simulink model "VBY_grid"  (R2024b)
settings: Solver=VariableStepAuto  StartTime=0.0  StopTime=24  MaxStep=0.33333333333333331  RelTol=1e-3  AbsTol=1e-3
values from neighbouring files (symbols this model uses):
  chargepower = 2E5    (= 200000)    [VBY_Script.m]
  terminalpower = 2E5    (= 200000)    [VBY_Script.m]
libraries: ee_lib x20, nesl_utility x16, fl_lib x10, simulink x8
settings Model: Creator=thoma  LastModifiedBy=thoma
settings SolverCC: AutoScaleAbsTol=off  DaesscMode=Robust
settings RTWCC: GenCodeOnly=on
settings SimscapeCC: SimscapeLogType=all

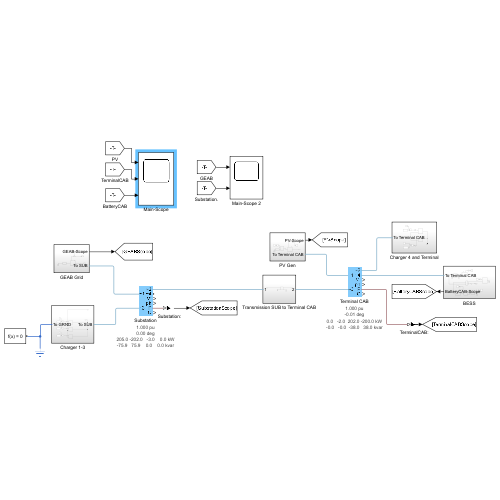
[thumbnail: Simulink's stored preview of the top-level diagram]
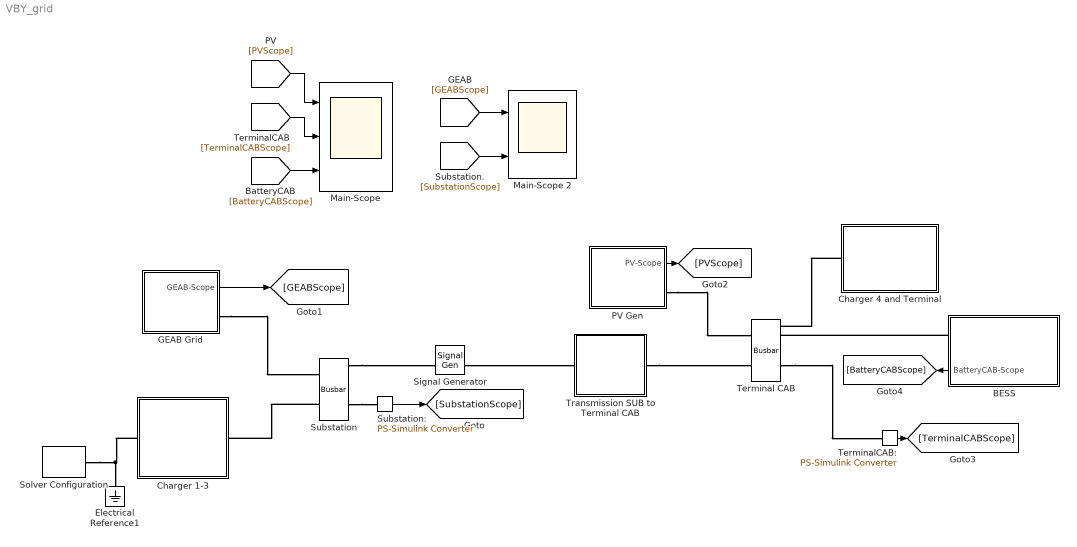
== system VBY_grid ==
  BESS : Subsystem
      settings: PortSchema="{\"entries\":[{\"content\":{\"sides\":[{\"content\":{\"connectorIds\":[\"LConn1\",\"Out1\"]},\"type\":\"ConnectorPlacement.EquallySpacedRectSide\",\"uuid\":\"78a52686-050b-473c-a829-dc142b2c03df\"},{\"content\":{\"side\":\"RIGHT\"},\"type\":\"ConnectorPlacement.EquallySpacedRectSide\",\"uuid\":\"16e0a1dc-1e2b-41fa-aa9e-07b8fe218401\"},{\"content\":{\"side\":\"TOP\"},\"type\":\"ConnectorPlacement.EquallySpacedRectSide\",\"uuid\":\"598e8960-ce00-4dd1-b062-18bc04a546a6\"}]},\"type\":\"ConnectorPlacement.EquallySpacedConnector\",\"uuid\":\"625199ba-0c11-4d67-98b2-801757f8b5e4\"}],\"packageUris\":[\"http://schema.mathworks.com/mf0/Connector/R2020b\"],\"version\":\"1.0\"}"
  Charger 1-3 : Subsystem
  Charger 4 and Terminal : Subsystem
  Electrical Reference1 : fl_lib/Electrical/Electrical Elements/Electrical Reference
  GEAB Grid : Subsystem
  Main-Scope : Scope  NumInputPorts=3
  Main-Scope 2 : Scope  NumInputPorts=2
  PV Gen : Subsystem
  Solver Configuration : nesl_utility/Solver Configuration  PhysicalDomain=network_engine_domain  SubClassName=solver  LeftPortType=input  RightPortType=generic  Tones=[]  Harmonics=[]  SimulateNoise=off  Profile=off  UseLocalSampling=off  EnableSwitchedLinearOptims=on  FrequencyDomain=off  UseCCode=off  RelTol=0.001  AbsTol=0.001  MinStep=1e-09  ToWorkspace=off  RevertToSquareIcSolve=off  NumHomotopyIterations=100  PhasorMode=off  PhasorModeNumHarmonics=1  ConsistencySolver=NEWTON_XTOL_AFTER_FTOL  IndexReductionMethod=DerivativeReplacement  DoDC=on  ResidualTolerance=1e-09  ConsistencyTolSource=GLOBAL  ConsistencyAbsTol=0.001  ConsistencyRelTol=0.001  ConsistencyTolFactor=0.0001  UseLocalSolver=off  LocalSolverChoice=NE_BACKWARD_EULER_ADVANCER  ResolveIndetEquations=on  FunctionEvalNumThread=1  LocalSolverSampleTime=0.001  DoFixedCost=off  MaxNonlinIter=3  MaxModeIter=2  ComputeImpulses=off  ImpulseIterations=2  LinearAlgebra=auto  LinearAlgebraNumThread=0  EquationFormulation=NE_FREQUENCY_TIME_EF  DelaysMemoryBudget=1024  AutomaticFiltering=on  FilteringTimeConstant=0.001  PartitionStorageMethod=AS_NEEDED  PartitionMemoryBudget=1024  PartitionMethod=ROBUST  MultibodyUseLocalSolver=off  MultibodyLocalSolverChoice=ODE1  MultibodyLocalSolverSampleTime=0.001
  Substation : ee_lib/Connectors & References/Busbar  Tag="1.000 pu\\n0.00 deg\\n205.0 -202.0   -3.0    0.0 kW\\n-75.9   75.9    0.0    0.0 kvar"  n_nodes=ee.enum.connectors.busbar_number_of_connections.four  VRated=11 kV  freq=50 Hz  show_ps=ee.enum.connectors.busbar_measurement.true
      settings: AttributesFormatString=%<Tag>  InternalSimscapePortConfiguration="{\"Bottom\":[],\"Left\":[{\"id\":\"N1\",\"label\":\"~1\",\"type\":\"foundation.electrical.three_phase\"},{\"id\":\"N3\",\"label\":\"~3\",\"type\":\"foundation.electrical.three_phase\"}],\"Right\":[{\"id\":\"N2\",\"label\":\"~2\",\"type\":\"foundation.electrical.three_phase\"},{\"id\":\"N4\",\"label\":\"~4\",\"type\":\"foundation.electrical.three_phase\"},{\"id\":\"Vt_ps\",\"label\":\"Vt\",\"type\":\"output\"},{\"id\":\"ph_ps\",\"label\":\"ph\",\"type\":\"output\"},{\"id\":\"P4_ps\",\"label\":\"P\",\"type\":\"output\"},{\"id\":\"Q4_ps\",\"label\":\"Q\",\"type\":\"output\"}],\"Top\":[]}"
  "Substation: " : nesl_utility/PS-Simulink Converter  PhysicalDomain=network_engine_domain  SubClassName=ps_output  LeftPortType=input  RightPortType=output  PseudoPeriodic=off  Frequencies=[]  VectorFormat=inherit  Unit=inherit  AffineConversion=off
  Terminal CAB : ee_lib/Connectors & References/Busbar  Tag="1.000 pu\\n-0.01 deg\\n0.0   -2.0  202.0 -200.0 kW\\n-0.0   -0.0  -38.0   38.0 kvar"  n_nodes=ee.enum.connectors.busbar_number_of_connections.four  VRated=11 kV  freq=50 Hz  show_ps=ee.enum.connectors.busbar_measurement.true
      settings: AttributesFormatString=%<Tag>  InternalSimscapePortConfiguration="{\"Bottom\":[],\"Left\":[{\"id\":\"N1\",\"label\":\"~1\",\"type\":\"foundation.electrical.three_phase\"},{\"id\":\"N3\",\"label\":\"~3\",\"type\":\"foundation.electrical.three_phase\"}],\"Right\":[{\"id\":\"N2\",\"label\":\"~2\",\"type\":\"foundation.electrical.three_phase\"},{\"id\":\"N4\",\"label\":\"~4\",\"type\":\"foundation.electrical.three_phase\"},{\"id\":\"Vt_ps\",\"label\":\"Vt\",\"type\":\"output\"},{\"id\":\"ph_ps\",\"label\":\"ph\",\"type\":\"output\"},{\"id\":\"P4_ps\",\"label\":\"P\",\"type\":\"output\"},{\"id\":\"Q4_ps\",\"label\":\"Q\",\"type\":\"output\"}],\"Top\":[]}"
  TerminalCAB: : nesl_utility/PS-Simulink Converter  PhysicalDomain=network_engine_domain  SubClassName=ps_output  LeftPortType=input  RightPortType=output  PseudoPeriodic=off  Frequencies=[]  VectorFormat=inherit  Unit=inherit  AffineConversion=off
  Transmission SUB to Terminal CAB : Subsystem
  Signal Generator : SignalGenerator  IOType=siggen
  wires:
  "Substation: "/1 -> [SubstationScope]
  GEAB Grid/1(GEAB-Scope) -> [GEABScope]
  PV Gen/1(PV-Scope) -> [PVScope]
  [PVScope] -> Main-Scope/1
  TerminalCAB:/1 -> [TerminalCABScope]
  [TerminalCABScope] -> Main-Scope/2
  BESS/1(BatteryCAB-Scope) -> [BatteryCABScope]
  [BatteryCABScope] -> Main-Scope/3
  [GEABScope] -> Main-Scope 2/1
  [SubstationScope] -> Main-Scope 2/2
  connections:
  Substation/RConn5 -- "Substation: "/LConn1
  Solver Configuration/RConn1 -- Charger 1-3/LConn1 -- Electrical Reference1/LConn1
  Substation/LConn2 -- Charger 1-3/RConn1
  BESS/LConn1 -- Terminal CAB/RConn2
  GEAB Grid/RConn1 -- Substation/LConn1
  PV Gen/RConn1 -- Terminal CAB/LConn1
  Charger 4 and Terminal/LConn1 -- Terminal CAB/RConn1
  Substation/RConn1 -- Transmission SUB to Terminal CAB/LConn1
  Transmission SUB to Terminal CAB/RConn1 -- Terminal CAB/LConn2
  Terminal CAB/RConn5 -- TerminalCAB:/LConn1

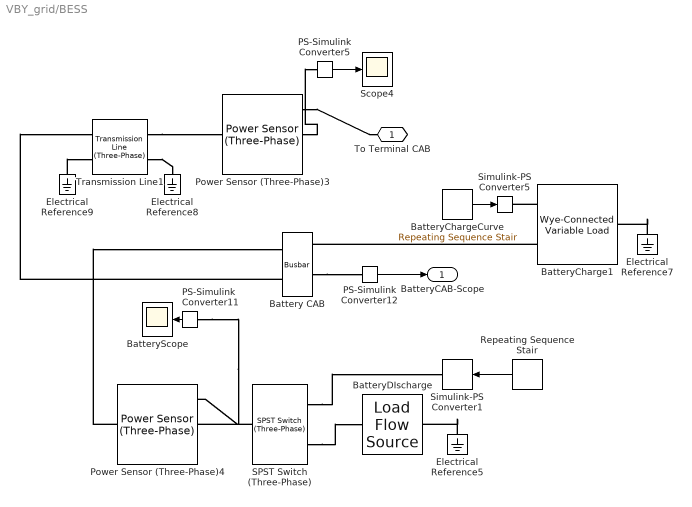
== system VBY_grid/BESS ==
  Battery CAB : ee_lib/Connectors & References/Busbar  Tag="1.000 pu\\n-0.02 deg\\n0.0 -200.0  200.0 kW\\n-0.0    0.0    0.0 kvar"  n_nodes=ee.enum.connectors.busbar_number_of_connections.three  VRated=11 kV  freq=50 Hz  show_ps=ee.enum.connectors.busbar_measurement.true
      settings: AttributesFormatString=%<Tag>  InternalSimscapePortConfiguration="{\"Bottom\":[],\"Left\":[{\"id\":\"N1\",\"label\":\"~1\",\"type\":\"foundation.electrical.three_phase\"},{\"id\":\"N3\",\"label\":\"~3\",\"type\":\"foundation.electrical.three_phase\"}],\"Right\":[{\"id\":\"N2\",\"label\":\"~2\",\"type\":\"foundation.electrical.three_phase\"},{\"id\":\"Vt_ps\",\"label\":\"Vt\",\"type\":\"output\"},{\"id\":\"ph_ps\",\"label\":\"ph\",\"type\":\"output\"},{\"id\":\"P3_ps\",\"label\":\"P\",\"type\":\"output\"},{\"id\":\"Q3_ps\",\"label\":\"Q\",\"type\":\"output\"}],\"Top\":[]}"
  BatteryCharge1 : ee_lib/Passive/RLC Assemblies/Wye-Connected Variable Load  VRated=11 kV  Pmin=1e3 W
      settings: InternalSimscapePortConfiguration="{\"Bottom\":[],\"Left\":[{\"id\":\"P\",\"label\":\"P\",\"type\":\"input\"},{\"id\":\"N\",\"label\":\"~\",\"type\":\"foundation.electrical.three_phase\"}],\"Right\":[{\"id\":\"n\",\"label\":\"n\",\"type\":\"foundation.electrical.electrical\"}],\"Top\":[]}"
  BatteryChargeCurve : simulink/Sources/Repeating Sequence Stair  OutValues=battery_charge_curve  tsamp=1  OutMin=[]  OutMax=[]  OutDataTypeStr=double  OutputDataTypeScalingMode=double  OutDataType=fixdt(0,8)  ConRadixGroup=Best Precision: Vector-wise  OutScaling=2^-12
  BatteryDIscharge : ee_lib/Sources/Load Flow Source  source_type=ee.enum.sources.load_flow_source_type.PV  v_pu_src=1  active_power_generated=batterydischarge W  active_power_consumed=0 W  reactive_power_consumed=0 A*V  v_pu=1.025  VRated=11 kV  freq=50 Hz  shift_src=0 deg  impedance_option=ee.enum.sources.load_flow_source_impedance.XRratio  SShortCircuit=330 MW  XR=15  R=0.01 Ohm  L=3.97e-4 H  G_parasitic=0 1/Ohm  minimum_pu=0.95  phase_search_range=[-30, 30] deg  I_specify=off  I_priority=None  I=[0, 0, 0] A  I_nominal_specify=off  I_nominal_value=1  I_nominal_unit=A  V_impedance_specify=off  V_impedance_priority=None  V_impedance=[0, 0, 0] V  V_impedance_nominal_specify=off  V_impedance_nominal_value=1  V_impedance_nominal_unit=V
      settings: InternalSimscapePortConfiguration="{\"Bottom\":[],\"Left\":[{\"id\":\"N\",\"label\":\"~\",\"type\":\"foundation.electrical.three_phase\"}],\"Right\":[{\"id\":\"n\",\"label\":\"n\",\"type\":\"foundation.electrical.electrical\"}],\"Top\":[]}"
  BatteryScope : Scope
  Electrical Reference{5,7..9} (4 alike) : fl_lib/Electrical/Electrical Elements/Electrical Reference
  PS-Simulink Converter11 : nesl_utility/PS-Simulink Converter  PhysicalDomain=network_engine_domain  SubClassName=ps_output  LeftPortType=input  RightPortType=output  PseudoPeriodic=off  Frequencies=[]  VectorFormat=inherit  Unit=inherit  AffineConversion=off
  PS-Simulink Converter12 : nesl_utility/PS-Simulink Converter  PhysicalDomain=network_engine_domain  SubClassName=ps_output  LeftPortType=input  RightPortType=output  PseudoPeriodic=off  Frequencies=[]  VectorFormat=inherit  Unit=inherit  AffineConversion=off
  PS-Simulink Converter5 : nesl_utility/PS-Simulink Converter  PhysicalDomain=network_engine_domain  SubClassName=ps_output  LeftPortType=input  RightPortType=output  PseudoPeriodic=off  Frequencies=[]  VectorFormat=inherit  Unit=inherit  AffineConversion=off
  Power Sensor (Three-Phase)3 : ee_lib/Sensors & Transducers/Power Sensor (Three-Phase)  load_type=ee.enum.passive.type_balanced.balanced  f0=50 Hz  config=ee.enum.with_neutral.no  rho=1
      settings: InternalSimscapePortConfiguration="{\"Bottom\":[],\"Left\":[{\"id\":\"N1\",\"label\":\"~1\",\"type\":\"foundation.electrical.three_phase\"}],\"Right\":[{\"id\":\"N2\",\"label\":\"~2\",\"type\":\"foundation.electrical.three_phase\"}],\"Top\":[{\"id\":\"Pm\",\"label\":\"P\",\"type\":\"output\"},{\"id\":\"Qm\",\"label\":\"Q\",\"type\":\"output\"}]}"
  Power Sensor (Three-Phase)4 : ee_lib/Sensors & Transducers/Power Sensor (Three-Phase)  load_type=ee.enum.passive.type_balanced.balanced  f0=50 Hz  config=ee.enum.with_neutral.no  rho=1
      settings: InternalSimscapePortConfiguration="{\"Bottom\":[],\"Left\":[{\"id\":\"N1\",\"label\":\"~1\",\"type\":\"foundation.electrical.three_phase\"}],\"Right\":[{\"id\":\"N2\",\"label\":\"~2\",\"type\":\"foundation.electrical.three_phase\"}],\"Top\":[{\"id\":\"Pm\",\"label\":\"P\",\"type\":\"output\"},{\"id\":\"Qm\",\"label\":\"Q\",\"type\":\"output\"}]}"
  Repeating Sequence Stair : simulink/Sources/Repeating Sequence Stair  OutValues=battery_power_curve  tsamp=1  OutMin=[]  OutMax=[]  OutDataTypeStr=double  OutputDataTypeScalingMode=double  OutDataType=fixdt(0,8)  ConRadixGroup=Best Precision: Vector-wise  OutScaling=2^-12
  SPST Switch (Three-Phase) : ee_lib/Switches & Breakers/SPST Switch (Three-Phase)  R_closed=0.001 Ohm  G_open=1e-6 1/Ohm  threshold=0.5 V  i_vT_specify=off  i_vT_priority=None  i_vT=0 A  i_vT_nominal_specify=off  i_vT_nominal_value=1  i_vT_nominal_unit=A  I_specify=off  I_priority=None  I=[0, 0, 0] A  I_nominal_specify=off  I_nominal_value=1  I_nominal_unit=A  V_specify=off  V_priority=None  V=[0, 0, 0] V  V_nominal_specify=off  V_nominal_value=1  V_nominal_unit=V  i_a_specify=off  i_a_priority=None  i_a=0 A  i_a_nominal_specify=off  i_a_nominal_value=1  i_a_nominal_unit=A  v_a_specify=off  v_a_priority=None  v_a=0 V  v_a_nominal_specify=off  v_a_nominal_value=1  v_a_nominal_unit=V  i_b_specify=off  i_b_priority=None  i_b=0 A  i_b_nominal_specify=off  i_b_nominal_value=1  i_b_nominal_unit=A  v_b_specify=off  v_b_priority=None  v_b=0 V  v_b_nominal_specify=off  v_b_nominal_value=1  v_b_nominal_unit=V  i_c_specify=off  i_c_priority=None  i_c=0 A  i_c_nominal_specify=off  i_c_nominal_value=1  i_c_nominal_unit=A  v_c_specify=off  v_c_priority=None  v_c=0 V  v_c_nominal_specify=off  v_c_nominal_value=1  v_c_nominal_unit=V
      settings: InternalSimscapePortConfiguration="{\"Bottom\":[],\"Left\":[{\"id\":\"vT\",\"label\":\"vT\",\"type\":\"input\"},{\"id\":\"N1\",\"label\":\"~1\",\"type\":\"foundation.electrical.three_phase\"}],\"Right\":[{\"id\":\"N2\",\"label\":\"~2\",\"type\":\"foundation.electrical.three_phase\"}],\"Top\":[]}"
  Scope4 : Scope
  Simulink-PS Converter1 : nesl_utility/Simulink-PS Converter  PhysicalDomain=network_engine_domain  SubClassName=ps_input  LeftPortType=input  RightPortType=output  PseudoPeriodic=off  Frequencies=[]  NoiseDistribution=none  NoiseParameters=[]  Unit=1  AffineConversion=off  FilteringAndDerivatives=filter  SimscapeFilterOrder=1  InputFilterTimeConstant=0.001  UdotUserProvided=0
  Simulink-PS Converter5 : nesl_utility/Simulink-PS Converter  PhysicalDomain=network_engine_domain  SubClassName=ps_input  LeftPortType=input  RightPortType=output  PseudoPeriodic=off  Frequencies=[]  NoiseDistribution=none  NoiseParameters=[]  Unit=1  AffineConversion=off  FilteringAndDerivatives=provide  SimscapeFilterOrder=1  InputFilterTimeConstant=0.001  UdotUserProvided=0
  Transmission Line1 : ee_lib/Passive/Lines/Transmission Line (Three-Phase)  length=1 km  freq=50 Hz  R=0.02 Ohm/km  L=0.5 mH/km  M=0.1 mH/km  Cl=0.3 uF/km  Cg=0.1 uF/km  Rm=0 Ohm/km  ModelTwoSections=ee.enum.enable.no  N=1  InterfacePosition=1 km  N1sec=1  N2sec=1  Access_ground=ee.enum.enable.no  R_parasitic=1e-6 Ohm  G_parasitic=1e-6 1/Ohm
      settings: InternalSimscapePortConfiguration="{\"Bottom\":[],\"Left\":[{\"id\":\"N1\",\"label\":\"~1\",\"type\":\"foundation.electrical.three_phase\"},{\"id\":\"g1\",\"label\":\"g1\",\"type\":\"foundation.electrical.electrical\"}],\"Right\":[{\"id\":\"N2\",\"label\":\"~2\",\"type\":\"foundation.electrical.three_phase\"},{\"id\":\"g2\",\"label\":\"g2\",\"type\":\"foundation.electrical.electrical\"}],\"Top\":[]}"
  To Terminal CAB : PMIOPort  Side=Left
  BatteryCAB-Scope : Outport
  wires:
  PS-Simulink Converter12/1 -> BatteryCAB-Scope/1
  PS-Simulink Converter5/1 -> Scope4/1
  BatteryChargeCurve/1 -> Simulink-PS Converter5/1
  PS-Simulink Converter11/1 -> BatteryScope/1
  Repeating Sequence Stair/1 -> Simulink-PS Converter1/1
  connections:
  Power Sensor (Three-Phase)4/RConn1 -- Battery CAB/LConn1
  Electrical Reference9/LConn1 -- Transmission Line1/LConn2
  Power Sensor (Three-Phase)3/LConn2 -- PS-Simulink Converter5/LConn1
  BatteryCharge1/LConn2 -- Battery CAB/RConn1
  Transmission Line1/RConn2 -- Electrical Reference8/LConn1
  Electrical Reference7/LConn1 -- BatteryCharge1/RConn1
  SPST Switch (Three-Phase)/RConn1 -- Power Sensor (Three-Phase)4/LConn1
  BatteryCharge1/LConn1 -- Simulink-PS Converter5/RConn1
  PS-Simulink Converter11/LConn1 -- Power Sensor (Three-Phase)4/LConn2
  Transmission Line1/RConn1 -- Power Sensor (Three-Phase)3/RConn1
  Battery CAB/LConn2 -- Transmission Line1/LConn1
  Electrical Reference5/LConn1 -- BatteryDIscharge/RConn1
  Battery CAB/RConn4 -- PS-Simulink Converter12/LConn1
  Power Sensor (Three-Phase)3/LConn1 -- To Terminal CAB/RConn1
  SPST Switch (Three-Phase)/LConn1 -- Simulink-PS Converter1/RConn1
  SPST Switch (Three-Phase)/LConn2 -- BatteryDIscharge/LConn1

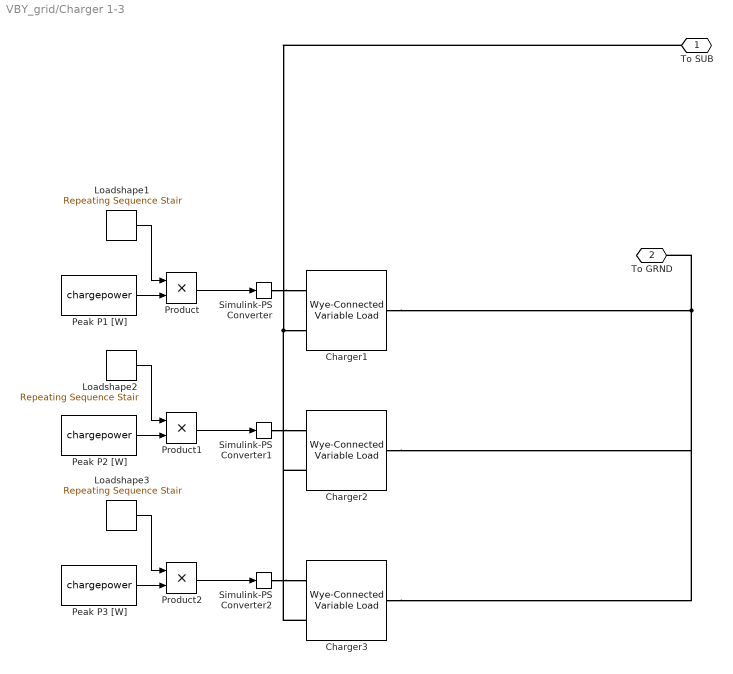
== system VBY_grid/Charger 1-3 ==
  Charger1 : ee_lib/Passive/RLC Assemblies/Wye-Connected Variable Load  VRated=11 kV  Pmin=1e3 W
      settings: InternalSimscapePortConfiguration="{\"Bottom\":[],\"Left\":[{\"id\":\"P\",\"label\":\"P\",\"type\":\"input\"},{\"id\":\"N\",\"label\":\"~\",\"type\":\"foundation.electrical.three_phase\"}],\"Right\":[{\"id\":\"n\",\"label\":\"n\",\"type\":\"foundation.electrical.electrical\"}],\"Top\":[]}"
  Charger2 : ee_lib/Passive/RLC Assemblies/Wye-Connected Variable Load  VRated=11 kV  Pmin=1e3 W
      settings: InternalSimscapePortConfiguration="{\"Bottom\":[],\"Left\":[{\"id\":\"P\",\"label\":\"P\",\"type\":\"input\"},{\"id\":\"N\",\"label\":\"~\",\"type\":\"foundation.electrical.three_phase\"}],\"Right\":[{\"id\":\"n\",\"label\":\"n\",\"type\":\"foundation.electrical.electrical\"}],\"Top\":[]}"
  Charger3 : ee_lib/Passive/RLC Assemblies/Wye-Connected Variable Load  VRated=11 kV  Pmin=1e3 W
      settings: InternalSimscapePortConfiguration="{\"Bottom\":[],\"Left\":[{\"id\":\"P\",\"label\":\"P\",\"type\":\"input\"},{\"id\":\"N\",\"label\":\"~\",\"type\":\"foundation.electrical.three_phase\"}],\"Right\":[{\"id\":\"n\",\"label\":\"n\",\"type\":\"foundation.electrical.electrical\"}],\"Top\":[]}"
  "Loadshape1 " : simulink/Sources/Repeating Sequence Stair  OutValues=loadshape1  tsamp=1  OutMin=[]  OutMax=[]  OutDataTypeStr=double  OutputDataTypeScalingMode=double  OutDataType=fixdt(0,8)  ConRadixGroup=Best Precision: Vector-wise  OutScaling=2^-12
  Loadshape2 : simulink/Sources/Repeating Sequence Stair  OutValues=loadshape2  tsamp=1  OutMin=[]  OutMax=[]  OutDataTypeStr=double  OutputDataTypeScalingMode=double  OutDataType=fixdt(0,8)  ConRadixGroup=Best Precision: Vector-wise  OutScaling=2^-12
  "Loadshape3 " : simulink/Sources/Repeating Sequence Stair  OutValues=loadshape3  tsamp=1  OutMin=[]  OutMax=[]  OutDataTypeStr=double  OutputDataTypeScalingMode=double  OutDataType=fixdt(0,8)  ConRadixGroup=Best Precision: Vector-wise  OutScaling=2^-12
  Peak P1 [W] : Constant  Value=chargepower
  Peak P2 [W] : Constant  Value=chargepower
  Peak P3 [W] : Constant  Value=chargepower
  Product : Product
  Product1 : Product
  Product2 : Product
  Simulink-PS Converter : nesl_utility/Simulink-PS Converter  PhysicalDomain=network_engine_domain  SubClassName=ps_input  LeftPortType=input  RightPortType=output  PseudoPeriodic=off  Frequencies=[]  NoiseDistribution=none  NoiseParameters=[]  Unit=1  AffineConversion=off  FilteringAndDerivatives=provide  SimscapeFilterOrder=1  InputFilterTimeConstant=0.001  UdotUserProvided=0
  Simulink-PS Converter1 : nesl_utility/Simulink-PS Converter  PhysicalDomain=network_engine_domain  SubClassName=ps_input  LeftPortType=input  RightPortType=output  PseudoPeriodic=off  Frequencies=[]  NoiseDistribution=none  NoiseParameters=[]  Unit=1  AffineConversion=off  FilteringAndDerivatives=provide  SimscapeFilterOrder=1  InputFilterTimeConstant=0.001  UdotUserProvided=0
  Simulink-PS Converter2 : nesl_utility/Simulink-PS Converter  PhysicalDomain=network_engine_domain  SubClassName=ps_input  LeftPortType=input  RightPortType=output  PseudoPeriodic=off  Frequencies=[]  NoiseDistribution=none  NoiseParameters=[]  Unit=1  AffineConversion=off  FilteringAndDerivatives=provide  SimscapeFilterOrder=1  InputFilterTimeConstant=0.001  UdotUserProvided=0
  To SUB : PMIOPort  Side=Right
  To GRND : PMIOPort  Port=2  Side=Left
  wires:
  Loadshape2/1 -> Product1/1
  Product/1 -> Simulink-PS Converter/1
  Peak P3 [W]/1 -> Product2/2
  Peak P2 [W]/1 -> Product1/2
  Peak P1 [W]/1 -> Product/2
  Product1/1 -> Simulink-PS Converter1/1
  "Loadshape1 "/1 -> Product/1
  "Loadshape3 "/1 -> Product2/1
  Product2/1 -> Simulink-PS Converter2/1
  connections:
  Simulink-PS Converter/RConn1 -- Charger1/LConn1
  Charger3/LConn2 -- Charger2/LConn2 -- To SUB/RConn1 -- Charger1/LConn2
  Charger3/RConn1 -- Charger2/RConn1 -- To GRND/RConn1 -- Charger1/RConn1
  Simulink-PS Converter1/RConn1 -- Charger2/LConn1
  Simulink-PS Converter2/RConn1 -- Charger3/LConn1

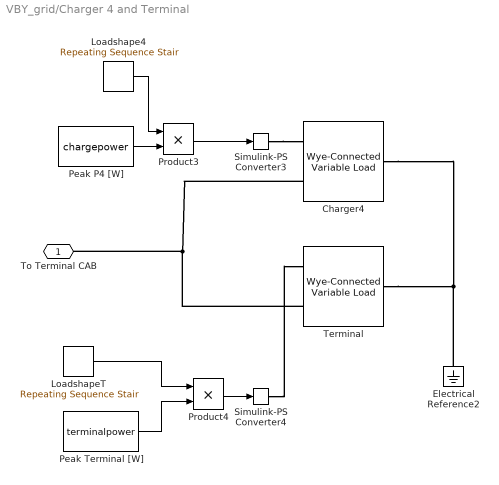
== system VBY_grid/Charger 4 and Terminal ==
  Charger4 : ee_lib/Passive/RLC Assemblies/Wye-Connected Variable Load  VRated=11 kV  Pmin=1e3 W
      settings: InternalSimscapePortConfiguration="{\"Bottom\":[],\"Left\":[{\"id\":\"P\",\"label\":\"P\",\"type\":\"input\"},{\"id\":\"N\",\"label\":\"~\",\"type\":\"foundation.electrical.three_phase\"}],\"Right\":[{\"id\":\"n\",\"label\":\"n\",\"type\":\"foundation.electrical.electrical\"}],\"Top\":[]}"
  Electrical Reference2 : fl_lib/Electrical/Electrical Elements/Electrical Reference
  Loadshape4 : simulink/Sources/Repeating Sequence Stair  OutValues=loadshape4  tsamp=1  OutMin=[]  OutMax=[]  OutDataTypeStr=double  OutputDataTypeScalingMode=double  OutDataType=fixdt(0,8)  ConRadixGroup=Best Precision: Vector-wise  OutScaling=2^-12
  LoadshapeT : simulink/Sources/Repeating Sequence Stair  OutValues=loadshapeT  tsamp=1  OutMin=[]  OutMax=[]  OutDataTypeStr=double  OutputDataTypeScalingMode=double  OutDataType=fixdt(0,8)  ConRadixGroup=Best Precision: Vector-wise  OutScaling=2^-12
  Peak P4 [W] : Constant  Value=chargepower
  Peak Terminal [W] : Constant  Value=terminalpower
  Product3 : Product
  Product4 : Product
  Simulink-PS Converter3 : nesl_utility/Simulink-PS Converter  PhysicalDomain=network_engine_domain  SubClassName=ps_input  LeftPortType=input  RightPortType=output  PseudoPeriodic=off  Frequencies=[]  NoiseDistribution=none  NoiseParameters=[]  Unit=1  AffineConversion=off  FilteringAndDerivatives=provide  SimscapeFilterOrder=1  InputFilterTimeConstant=0.001  UdotUserProvided=0
  Simulink-PS Converter4 : nesl_utility/Simulink-PS Converter  PhysicalDomain=network_engine_domain  SubClassName=ps_input  LeftPortType=input  RightPortType=output  PseudoPeriodic=off  Frequencies=[]  NoiseDistribution=none  NoiseParameters=[]  Unit=1  AffineConversion=off  FilteringAndDerivatives=provide  SimscapeFilterOrder=1  InputFilterTimeConstant=0.001  UdotUserProvided=0
  Terminal : ee_lib/Passive/RLC Assemblies/Wye-Connected Variable Load  VRated=11 kV  Pmin=1e3 W
      settings: InternalSimscapePortConfiguration="{\"Bottom\":[],\"Left\":[{\"id\":\"P\",\"label\":\"P\",\"type\":\"input\"},{\"id\":\"N\",\"label\":\"~\",\"type\":\"foundation.electrical.three_phase\"}],\"Right\":[{\"id\":\"n\",\"label\":\"n\",\"type\":\"foundation.electrical.electrical\"}],\"Top\":[]}"
  To Terminal CAB : PMIOPort  Side=Left
  wires:
  Loadshape4/1 -> Product3/1
  Product4/1 -> Simulink-PS Converter4/1
  Product3/1 -> Simulink-PS Converter3/1
  Peak Terminal [W]/1 -> Product4/2
  Peak P4 [W]/1 -> Product3/2
  LoadshapeT/1 -> Product4/1
  connections:
  Simulink-PS Converter4/RConn1 -- Terminal/LConn1
  Simulink-PS Converter3/RConn1 -- Charger4/LConn1
  Electrical Reference2/LConn1 -- Charger4/RConn1 -- Terminal/RConn1
  Terminal/LConn2 -- Charger4/LConn2 -- To Terminal CAB/RConn1

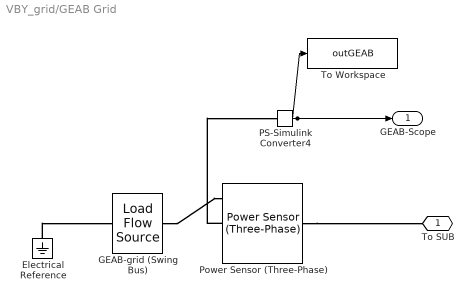
== system VBY_grid/GEAB Grid ==
  Electrical Reference : fl_lib/Electrical/Electrical Elements/Electrical Reference
  GEAB-grid (Swing Bus) : ee_lib/Sources/Load Flow Source  source_type=ee.enum.sources.load_flow_source_type.Swing  v_pu_src=1  active_power_generated=1.5 MW  active_power_consumed=0 W  reactive_power_consumed=0 A*V  v_pu=1  VRated=11 kV  freq=50 Hz  shift_src=0 deg  impedance_option=ee.enum.sources.load_flow_source_impedance.None  SShortCircuit=10 MW  XR=15  R=0.01 Ohm  L=3.97e-4 H  G_parasitic=0 1/Ohm  minimum_pu=0.95  phase_search_range=[-30, 30] deg  I_specify=off  I_priority=None  I=[0, 0, 0] A  I_nominal_specify=off  I_nominal_value=1  I_nominal_unit=A  V_impedance_specify=off  V_impedance_priority=None  V_impedance=[0, 0, 0] V  V_impedance_nominal_specify=off  V_impedance_nominal_value=1  V_impedance_nominal_unit=V
      settings: InternalSimscapePortConfiguration="{\"Bottom\":[],\"Left\":[{\"id\":\"N\",\"label\":\"~\",\"type\":\"foundation.electrical.three_phase\"}],\"Right\":[{\"id\":\"n\",\"label\":\"n\",\"type\":\"foundation.electrical.electrical\"}],\"Top\":[]}"
  PS-Simulink Converter4 : nesl_utility/PS-Simulink Converter  PhysicalDomain=network_engine_domain  SubClassName=ps_output  LeftPortType=input  RightPortType=output  PseudoPeriodic=off  Frequencies=[]  VectorFormat=inherit  Unit=inherit  AffineConversion=off
  Power Sensor (Three-Phase) : ee_lib/Sensors & Transducers/Power Sensor (Three-Phase)  load_type=ee.enum.passive.type_balanced.balanced  f0=60 Hz  config=ee.enum.with_neutral.no  rho=1
      settings: InternalSimscapePortConfiguration="{\"Bottom\":[],\"Left\":[{\"id\":\"N1\",\"label\":\"~1\",\"type\":\"foundation.electrical.three_phase\"}],\"Right\":[{\"id\":\"N2\",\"label\":\"~2\",\"type\":\"foundation.electrical.three_phase\"}],\"Top\":[{\"id\":\"Pm\",\"label\":\"P\",\"type\":\"output\"},{\"id\":\"Qm\",\"label\":\"Q\",\"type\":\"output\"}]}"
  To Workspace : ToWorkspace  VariableName=outGEAB  SampleTime=1
  To SUB : PMIOPort  Side=Right
  GEAB-Scope : Outport
  wires:
  PS-Simulink Converter4/1 -> GEAB-Scope/1, To Workspace/1
  connections:
  Power Sensor (Three-Phase)/LConn2 -- PS-Simulink Converter4/LConn1
  Electrical Reference/LConn1 -- GEAB-grid (Swing Bus)/RConn1
  Power Sensor (Three-Phase)/RConn1 -- To SUB/RConn1
  GEAB-grid (Swing Bus)/LConn1 -- Power Sensor (Three-Phase)/LConn1

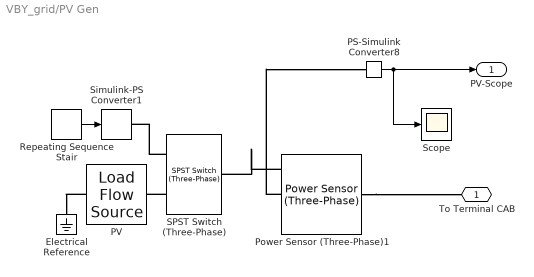
== system VBY_grid/PV Gen ==
  Electrical Reference : fl_lib/Electrical/Electrical Elements/Electrical Reference
  PS-Simulink Converter8 : nesl_utility/PS-Simulink Converter  PhysicalDomain=network_engine_domain  SubClassName=ps_output  LeftPortType=input  RightPortType=output  PseudoPeriodic=off  Frequencies=[]  VectorFormat=inherit  Unit=inherit  AffineConversion=off
  PV : ee_lib/Sources/Load Flow Source  source_type=ee.enum.sources.load_flow_source_type.PV  v_pu_src=1  active_power_generated=solarpower W  active_power_consumed=0 W  reactive_power_consumed=0 A*V  v_pu=1.025  VRated=11 kV  freq=50 Hz  shift_src=0 deg  impedance_option=ee.enum.sources.load_flow_source_impedance.XRratio  SShortCircuit=600 MW  XR=15  R=0.01 Ohm  L=3.97e-4 H  G_parasitic=0 1/Ohm  minimum_pu=0.95  phase_search_range=[-30,30] deg  I_specify=off  I_priority=None  I=[0, 0, 0] A  I_nominal_specify=off  I_nominal_value=1  I_nominal_unit=A  V_impedance_specify=off  V_impedance_priority=None  V_impedance=[0, 0, 0] V  V_impedance_nominal_specify=off  V_impedance_nominal_value=1  V_impedance_nominal_unit=V
      settings: InternalSimscapePortConfiguration="{\"Bottom\":[],\"Left\":[{\"id\":\"N\",\"label\":\"~\",\"type\":\"foundation.electrical.three_phase\"}],\"Right\":[{\"id\":\"n\",\"label\":\"n\",\"type\":\"foundation.electrical.electrical\"}],\"Top\":[]}"
  Power Sensor (Three-Phase)1 : ee_lib/Sensors & Transducers/Power Sensor (Three-Phase)  load_type=ee.enum.passive.type_balanced.balanced  f0=50 Hz  config=ee.enum.with_neutral.no  rho=1
      settings: InternalSimscapePortConfiguration="{\"Bottom\":[],\"Left\":[{\"id\":\"N1\",\"label\":\"~1\",\"type\":\"foundation.electrical.three_phase\"}],\"Right\":[{\"id\":\"N2\",\"label\":\"~2\",\"type\":\"foundation.electrical.three_phase\"}],\"Top\":[{\"id\":\"Pm\",\"label\":\"P\",\"type\":\"output\"},{\"id\":\"Qm\",\"label\":\"Q\",\"type\":\"output\"}]}"
  Repeating Sequence Stair : simulink/Sources/Repeating Sequence Stair  OutValues=solar_power_curve  tsamp=1  OutMin=[]  OutMax=[]  OutDataTypeStr=double  OutputDataTypeScalingMode=double  OutDataType=fixdt(0,8)  ConRadixGroup=Best Precision: Vector-wise  OutScaling=2^-12
  SPST Switch (Three-Phase) : ee_lib/Switches & Breakers/SPST Switch (Three-Phase)  R_closed=0.001 Ohm  G_open=1e-6 1/Ohm  threshold=0.5 V  i_vT_specify=off  i_vT_priority=None  i_vT=0 A  i_vT_nominal_specify=off  i_vT_nominal_value=1  i_vT_nominal_unit=A  I_specify=off  I_priority=None  I=[0, 0, 0] A  I_nominal_specify=off  I_nominal_value=1  I_nominal_unit=A  V_specify=off  V_priority=None  V=[0, 0, 0] V  V_nominal_specify=off  V_nominal_value=1  V_nominal_unit=V  i_a_specify=off  i_a_priority=None  i_a=0 A  i_a_nominal_specify=off  i_a_nominal_value=1  i_a_nominal_unit=A  v_a_specify=off  v_a_priority=None  v_a=0 V  v_a_nominal_specify=off  v_a_nominal_value=1  v_a_nominal_unit=V  i_b_specify=off  i_b_priority=None  i_b=0 A  i_b_nominal_specify=off  i_b_nominal_value=1  i_b_nominal_unit=A  v_b_specify=off  v_b_priority=None  v_b=0 V  v_b_nominal_specify=off  v_b_nominal_value=1  v_b_nominal_unit=V  i_c_specify=off  i_c_priority=None  i_c=0 A  i_c_nominal_specify=off  i_c_nominal_value=1  i_c_nominal_unit=A  v_c_specify=off  v_c_priority=None  v_c=0 V  v_c_nominal_specify=off  v_c_nominal_value=1  v_c_nominal_unit=V
      settings: InternalSimscapePortConfiguration="{\"Bottom\":[],\"Left\":[{\"id\":\"vT\",\"label\":\"vT\",\"type\":\"input\"},{\"id\":\"N1\",\"label\":\"~1\",\"type\":\"foundation.electrical.three_phase\"}],\"Right\":[{\"id\":\"N2\",\"label\":\"~2\",\"type\":\"foundation.electrical.three_phase\"}],\"Top\":[]}"
  Scope : Scope
  Simulink-PS Converter1 : nesl_utility/Simulink-PS Converter  PhysicalDomain=network_engine_domain  SubClassName=ps_input  LeftPortType=input  RightPortType=output  PseudoPeriodic=off  Frequencies=[]  NoiseDistribution=none  NoiseParameters=[]  Unit=1  AffineConversion=off  FilteringAndDerivatives=filter  SimscapeFilterOrder=1  InputFilterTimeConstant=0.001  UdotUserProvided=0
  To Terminal CAB : PMIOPort  Side=Right
  PV-Scope : Outport
  wires:
  PS-Simulink Converter8/1 -> Scope/1, PV-Scope/1
  Repeating Sequence Stair/1 -> Simulink-PS Converter1/1
  connections:
  Power Sensor (Three-Phase)1/LConn2 -- PS-Simulink Converter8/LConn1
  Power Sensor (Three-Phase)1/RConn1 -- To Terminal CAB/RConn1
  PV/RConn1 -- Electrical Reference/LConn1
  SPST Switch (Three-Phase)/LConn2 -- PV/LConn1
  SPST Switch (Three-Phase)/LConn1 -- Simulink-PS Converter1/RConn1
  Power Sensor (Three-Phase)1/LConn1 -- SPST Switch (Three-Phase)/RConn1

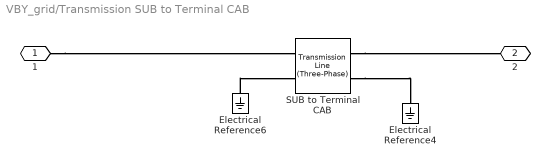
== system VBY_grid/Transmission SUB to Terminal CAB ==
  " SUB to Terminal CAB" : ee_lib/Passive/Lines/Transmission Line (Three-Phase)  length=1 km  freq=50 Hz  R=0.02 Ohm/km  L=0.5 mH/km  M=0.1 mH/km  Cl=0.3 uF/km  Cg=0.1 uF/km  Rm=0 Ohm/km  ModelTwoSections=ee.enum.enable.no  N=1  InterfacePosition=1 km  N1sec=1  N2sec=1  Access_ground=ee.enum.enable.no  R_parasitic=1e-6 Ohm  G_parasitic=1e-6 1/Ohm
      settings: InternalSimscapePortConfiguration="{\"Bottom\":[],\"Left\":[{\"id\":\"N1\",\"label\":\"~1\",\"type\":\"foundation.electrical.three_phase\"},{\"id\":\"g1\",\"label\":\"g1\",\"type\":\"foundation.electrical.electrical\"}],\"Right\":[{\"id\":\"N2\",\"label\":\"~2\",\"type\":\"foundation.electrical.three_phase\"},{\"id\":\"g2\",\"label\":\"g2\",\"type\":\"foundation.electrical.electrical\"}],\"Top\":[]}"
  Electrical Reference4 : fl_lib/Electrical/Electrical Elements/Electrical Reference
  Electrical Reference6 : fl_lib/Electrical/Electrical Elements/Electrical Reference
  1 : PMIOPort  Side=Left
  2 : PMIOPort  Port=2  Side=Right
  connections:
  1/RConn1 -- " SUB to Terminal CAB"/LConn1
  Electrical Reference6/LConn1 -- " SUB to Terminal CAB"/LConn2
  " SUB to Terminal CAB"/RConn2 -- Electrical Reference4/LConn1
  " SUB to Terminal CAB"/RConn1 -- 2/RConn1
